simulink model "PWMModel"  (R2025a)
settings: Solver=ode45  StartTime=0.0  StopTime=10  MaxStep=0.001  MinStep=0.0001  RelTol=1e-3
libraries: simulink x1
settings Model: DataDictionary=Constants.sldd  Creator=Alex V  LastModifiedBy=yaremadzulynsky

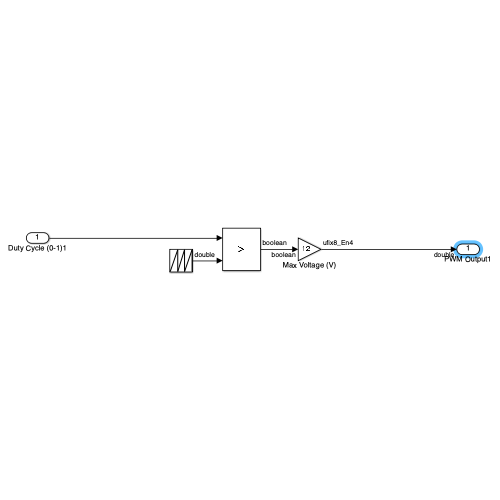
[thumbnail: Simulink's stored preview of the top-level diagram]
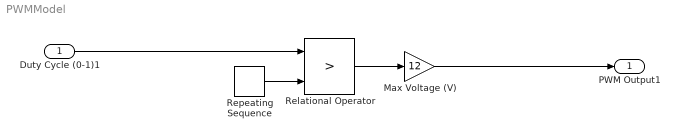
== system PWMModel ==
  Duty Cycle (0-1)1 : Inport  SampleTime=0
  Max Voltage (V) : Gain  Gain=12  OutDataTypeStr=double
  Relational Operator : RelationalOperator  Operator=>  OutDataTypeStr=boolean  RndMeth=Simplest  InputSameDT=off
  Repeating Sequence : simulink/Sources/Repeating Sequence  rep_seq_t=[0 0.1]  rep_seq_y=[0 1]
  PWM Output1 : Outport
  wires:
  Max Voltage (V)/1 -> PWM Output1/1
  Duty Cycle (0-1)1/1 -> Relational Operator/1
  Relational Operator/1 -> Max Voltage (V)/1
  Repeating Sequence/1 -> Relational Operator/2
